simulink model "Hinfinitysimulink"  (R2021a)
settings: Solver=VariableStepAuto  StartTime=0.0  StopTime=10.0  MaxStep=1e-4  RelTol=1e-3
values from neighbouring files (symbols this model uses):
  Aa_m = [0 1 0 ... (first row only)    [H_INFINITY_FINAL.m]
  Aaa_m = [-100500 1 0 ... (first row only)    [H_INFINITY_FINAL.m]
  Bb_m = [0 0 ... (first row only)    [H_INFINITY_FINAL.m]
  Bbb_m = [-100500 0 ... (first row only)    [H_INFINITY_FINAL.m]
  Cc_m = [-1 0 0 ... (first row only)    [H_INFINITY_FINAL.m]
  Ccc_m = [25420000000 1423000 -1331 ... (first row only)    [H_INFINITY_FINAL.m]
  Dd_m = [0 0 ... (first row only)    [H_INFINITY_FINAL.m]
  Ddd_m = [0 0 ... (first row only)    [H_INFINITY_FINAL.m]
settings Model: Creator=ANIRUDH  LastModifiedBy=ANIRUDH
settings SolverCC: AlgebraicLoopSolver=TrustRegion
settings DebuggingCC: SFMachineParentedDataDiag=warning
settings SFSimCC: CustomCodeUndefinedFunction=UseInterfaceOnly

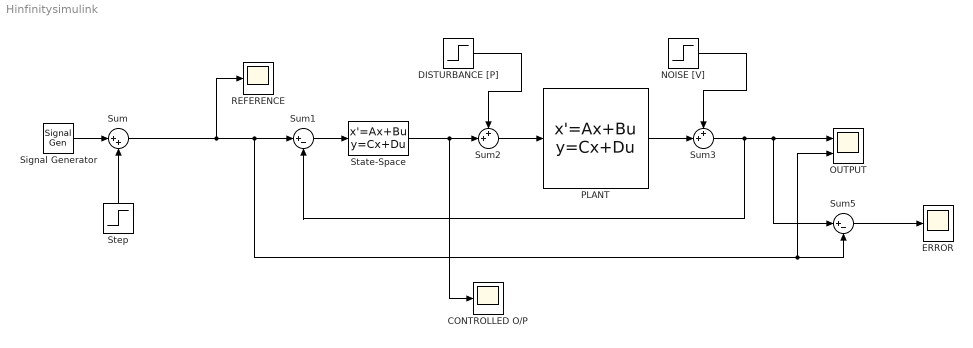
== system Hinfinitysimulink ==
  CONTROLLED O/P : Scope
  DISTURBANCE [P] : Step  Time=0  After=0  SampleTime=0
  ERROR : Scope
  NOISE [V] : Step  Time=0  After=0  SampleTime=0
  OUTPUT : Scope  NumInputPorts=2
  PLANT : StateSpace  A=Aa_m  B=Bb_m  C=Cc_m  D=Dd_m  InitialCondition=0  AllowTunableDMatrix=on
  REFERENCE : Scope
  Signal Generator : SignalGenerator  Amplitude=0.0000000000002  Frequency=0.000000000010  Units=rad/sec
  State-Space : StateSpace  A=Aaa_m  B=Bbb_m  C=Ccc_m  D=Ddd_m  InitialCondition=0  AllowTunableDMatrix=on
  Step : Step  Time=0  After=2  SampleTime=0
  Sum : Sum  Inputs=|++
  Sum1 : Sum  Inputs=|+-
  Sum2 : Sum  Inputs=++|
  Sum3 : Sum  Inputs=++|
  Sum5 : Sum  Inputs=|+-
  wires:
  Sum1/1 -> State-Space/1
  Sum2/1 -> PLANT/1
  State-Space/1 -> Sum2/2, CONTROLLED O/P/1
  NOISE [V]/1 -> Sum3/1
  PLANT/1 -> Sum3/2
  Sum/1 -> Sum5/2, OUTPUT/2, Sum1/1, REFERENCE/1
  DISTURBANCE [P]/1 -> Sum2/1
  Sum5/1 -> ERROR/1
  Step/1 -> Sum/2
  Signal Generator/1 -> Sum/1
  Sum3/1 -> Sum1/2, OUTPUT/1, Sum5/1
